simulink model "14_bus"  (R2024a)
settings: Solver=VariableStepAuto  StartTime=0.0  StopTime=1  RelTol=1e-3
undefined symbols (not defined in the file): D1, Delta
libraries: spsRMSLib x186, simulink_extras x171, spsThreePhaseVIMeasurementLib x94, spsThreePhaseBreakerLib x62, spsThreePhaseSeriesRLCBranchLib x20, spsThreePhaseSeriesRLCLoadLib x12, spsThreePhaseSourceLib x5, spsLoadFlowBusLib x5, spsStairGeneratorLib x5, spsThreePhaseTransformerTwoWindingsLib x5, spsThreePhaseFaultLib x5, sps_lib x1
(part 4 of 6)

== system 14_bus/Subsystem14/Subsystem22 ==
  Iabc1 : Inport
  Constant : Constant  Value=2  OutDataTypeStr=boolean
  Constant1 : Constant  Value=0  OutDataTypeStr=boolean
  Data Type Conversion : DataTypeConversion  OutDataTypeStr=double  SaturateOnIntegerOverflow=off  RndMeth=Floor
  Demux : Demux  Outputs=3
  Logical Operator : Logic  Inputs=3  AllPortsSameDT=off  OutDataTypeStr=boolean
  RMS : spsRMSLib/RMS  TrueRMS=on  Freq=60  RMSInit=120  Ts=0
  RMS1 : spsRMSLib/RMS  TrueRMS=on  Freq=60  RMSInit=120  Ts=0
  RMS2 : spsRMSLib/RMS  TrueRMS=on  Freq=60  RMSInit=120  Ts=0
  Relational Operator : RelationalOperator  Operator=>  OutDataTypeStr=boolean  RndMeth=Simplest  InputSameDT=off
  Relational Operator1 : RelationalOperator  Operator=>  OutDataTypeStr=boolean  RndMeth=Simplest  InputSameDT=off
  Relational Operator2 : RelationalOperator  Operator=>  OutDataTypeStr=boolean  RndMeth=Simplest  InputSameDT=off
  S-R Flip-Flop : simulink_extras/Flip Flops/S-R Flip-Flop  initial_condition=0
  S-R Flip-Flop1 : simulink_extras/Flip Flops/S-R Flip-Flop  initial_condition=0
  S-R Flip-Flop2 : simulink_extras/Flip Flops/S-R Flip-Flop  initial_condition=0
  Terminator : Terminator
  Terminator1 : Terminator
  Terminator2 : Terminator
  Out1 : Outport
  wires:
  Data Type Conversion/1 -> Out1/1
  Relational Operator/1 -> S-R Flip-Flop/1
  Constant1/1 -> S-R Flip-Flop/2, S-R Flip-Flop1/2, S-R Flip-Flop2/2
  RMS/1 -> Relational Operator/1
  S-R Flip-Flop1/2 -> Terminator1/1
  S-R Flip-Flop/2 -> Terminator/1
  S-R Flip-Flop2/2 -> Terminator2/1
  Iabc1/1 -> Demux/1
  Logical Operator/1 -> Data Type Conversion/1
  Constant/1 -> Relational Operator/2, Relational Operator1/2, Relational Operator2/2
  S-R Flip-Flop2/1 -> Logical Operator/3
  Relational Operator1/1 -> S-R Flip-Flop1/1
  S-R Flip-Flop/1 -> Logical Operator/1
  S-R Flip-Flop1/1 -> Logical Operator/2
  Relational Operator2/1 -> S-R Flip-Flop2/1
  Demux/1 -> RMS/1
  RMS2/1 -> Relational Operator1/1
  Demux/2 -> RMS2/1
  RMS1/1 -> Relational Operator2/1
  Demux/3 -> RMS1/1

== system 14_bus/Subsystem15/Subsystem8 ==
  Iabc1 : Inport
  Constant : Constant  Value=2  OutDataTypeStr=boolean
  Constant1 : Constant  Value=0  OutDataTypeStr=boolean
  Data Type Conversion : DataTypeConversion  OutDataTypeStr=double  SaturateOnIntegerOverflow=off  RndMeth=Floor
  Demux : Demux  Outputs=3
  Logical Operator : Logic  Inputs=3  AllPortsSameDT=off  OutDataTypeStr=boolean
  RMS : spsRMSLib/RMS  TrueRMS=on  Freq=60  RMSInit=120  Ts=0
  RMS1 : spsRMSLib/RMS  TrueRMS=on  Freq=60  RMSInit=120  Ts=0
  RMS2 : spsRMSLib/RMS  TrueRMS=on  Freq=60  RMSInit=120  Ts=0
  Relational Operator : RelationalOperator  Operator=>  OutDataTypeStr=boolean  RndMeth=Simplest  InputSameDT=off
  Relational Operator1 : RelationalOperator  Operator=>  OutDataTypeStr=boolean  RndMeth=Simplest  InputSameDT=off
  Relational Operator2 : RelationalOperator  Operator=>  OutDataTypeStr=boolean  RndMeth=Simplest  InputSameDT=off
  S-R Flip-Flop : simulink_extras/Flip Flops/S-R Flip-Flop  initial_condition=0
  S-R Flip-Flop1 : simulink_extras/Flip Flops/S-R Flip-Flop  initial_condition=0
  S-R Flip-Flop2 : simulink_extras/Flip Flops/S-R Flip-Flop  initial_condition=0
  Terminator : Terminator
  Terminator1 : Terminator
  Terminator2 : Terminator
  Out1 : Outport
  wires:
  Data Type Conversion/1 -> Out1/1
  Relational Operator/1 -> S-R Flip-Flop/1
  Constant1/1 -> S-R Flip-Flop/2, S-R Flip-Flop1/2, S-R Flip-Flop2/2
  RMS/1 -> Relational Operator/1
  S-R Flip-Flop1/2 -> Terminator1/1
  S-R Flip-Flop/2 -> Terminator/1
  S-R Flip-Flop2/2 -> Terminator2/1
  Iabc1/1 -> Demux/1
  Logical Operator/1 -> Data Type Conversion/1
  Constant/1 -> Relational Operator/2, Relational Operator1/2, Relational Operator2/2
  S-R Flip-Flop2/1 -> Logical Operator/3
  Relational Operator1/1 -> S-R Flip-Flop1/1
  S-R Flip-Flop/1 -> Logical Operator/1
  S-R Flip-Flop1/1 -> Logical Operator/2
  Relational Operator2/1 -> S-R Flip-Flop2/1
  Demux/1 -> RMS/1
  RMS1/1 -> Relational Operator1/1
  Demux/2 -> RMS1/1
  RMS2/1 -> Relational Operator2/1
  Demux/3 -> RMS2/1

== system 14_bus/Subsystem16/Subsystem15 ==
  Iabc1 : Inport
  Constant : Constant  Value=2  OutDataTypeStr=boolean
  Constant1 : Constant  Value=0  OutDataTypeStr=boolean
  Data Type Conversion : DataTypeConversion  OutDataTypeStr=double  SaturateOnIntegerOverflow=off  RndMeth=Floor
  Demux : Demux  Outputs=3
  Logical Operator : Logic  Inputs=3  AllPortsSameDT=off  OutDataTypeStr=boolean
  RMS : spsRMSLib/RMS  TrueRMS=on  Freq=60  RMSInit=120  Ts=0
  RMS1 : spsRMSLib/RMS  TrueRMS=on  Freq=60  RMSInit=120  Ts=0
  RMS2 : spsRMSLib/RMS  TrueRMS=on  Freq=60  RMSInit=120  Ts=0
  Relational Operator : RelationalOperator  Operator=>  OutDataTypeStr=boolean  RndMeth=Simplest  InputSameDT=off
  Relational Operator1 : RelationalOperator  Operator=>  OutDataTypeStr=boolean  RndMeth=Simplest  InputSameDT=off
  Relational Operator2 : RelationalOperator  Operator=>  OutDataTypeStr=boolean  RndMeth=Simplest  InputSameDT=off
  S-R Flip-Flop : simulink_extras/Flip Flops/S-R Flip-Flop  initial_condition=0
  S-R Flip-Flop1 : simulink_extras/Flip Flops/S-R Flip-Flop  initial_condition=0
  S-R Flip-Flop2 : simulink_extras/Flip Flops/S-R Flip-Flop  initial_condition=0
  Terminator : Terminator
  Terminator1 : Terminator
  Terminator2 : Terminator
  Out1 : Outport
  wires:
  Data Type Conversion/1 -> Out1/1
  Relational Operator/1 -> S-R Flip-Flop/1
  Constant1/1 -> S-R Flip-Flop/2, S-R Flip-Flop1/2, S-R Flip-Flop2/2
  RMS/1 -> Relational Operator/1
  S-R Flip-Flop1/2 -> Terminator1/1
  S-R Flip-Flop/2 -> Terminator/1
  S-R Flip-Flop2/2 -> Terminator2/1
  Iabc1/1 -> Demux/1
  Logical Operator/1 -> Data Type Conversion/1
  Constant/1 -> Relational Operator/2, Relational Operator1/2, Relational Operator2/2
  S-R Flip-Flop2/1 -> Logical Operator/3
  Relational Operator1/1 -> S-R Flip-Flop1/1
  S-R Flip-Flop/1 -> Logical Operator/1
  S-R Flip-Flop1/1 -> Logical Operator/2
  Relational Operator2/1 -> S-R Flip-Flop2/1
  Demux/1 -> RMS/1
  RMS1/1 -> Relational Operator1/1
  Demux/2 -> RMS1/1
  ? -> Relational Operator2/1
  Demux/3 -> RMS2/1

== system 14_bus/Subsystem17/Subsystem1 ==
  Iabc1 : Inport
  Constant : Constant  Value=2  OutDataTypeStr=boolean
  Constant1 : Constant  Value=0  OutDataTypeStr=boolean
  Data Type Conversion : DataTypeConversion  OutDataTypeStr=double  SaturateOnIntegerOverflow=off  RndMeth=Floor
  Demux : Demux  Outputs=3
  Logical Operator : Logic  Inputs=3  AllPortsSameDT=off  OutDataTypeStr=boolean
  RMS : spsRMSLib/RMS  TrueRMS=on  Freq=60  RMSInit=120  Ts=0
  RMS1 : spsRMSLib/RMS  TrueRMS=on  Freq=60  RMSInit=120  Ts=0
  RMS2 : spsRMSLib/RMS  TrueRMS=on  Freq=60  RMSInit=120  Ts=0
  Relational Operator : RelationalOperator  Operator=>  OutDataTypeStr=boolean  RndMeth=Simplest  InputSameDT=off
  Relational Operator1 : RelationalOperator  Operator=>  OutDataTypeStr=boolean  RndMeth=Simplest  InputSameDT=off
  Relational Operator2 : RelationalOperator  Operator=>  OutDataTypeStr=boolean  RndMeth=Simplest  InputSameDT=off
  S-R Flip-Flop : simulink_extras/Flip Flops/S-R Flip-Flop  initial_condition=0
  S-R Flip-Flop1 : simulink_extras/Flip Flops/S-R Flip-Flop  initial_condition=0
  S-R Flip-Flop2 : simulink_extras/Flip Flops/S-R Flip-Flop  initial_condition=0
  Terminator : Terminator
  Terminator1 : Terminator
  Terminator2 : Terminator
  Out1 : Outport
  wires:
  Data Type Conversion/1 -> Out1/1
  Relational Operator/1 -> S-R Flip-Flop/1
  Constant1/1 -> S-R Flip-Flop/2, S-R Flip-Flop1/2, S-R Flip-Flop2/2
  RMS/1 -> Relational Operator/1
  S-R Flip-Flop1/2 -> Terminator1/1
  S-R Flip-Flop/2 -> Terminator/1
  S-R Flip-Flop2/2 -> Terminator2/1
  Iabc1/1 -> Demux/1
  Logical Operator/1 -> Data Type Conversion/1
  Constant/1 -> Relational Operator/2, Relational Operator1/2, Relational Operator2/2
  S-R Flip-Flop2/1 -> Logical Operator/3
  Relational Operator1/1 -> S-R Flip-Flop1/1
  S-R Flip-Flop/1 -> Logical Operator/1
  S-R Flip-Flop1/1 -> Logical Operator/2
  Relational Operator2/1 -> S-R Flip-Flop2/1
  Demux/1 -> RMS/1
  RMS1/1 -> Relational Operator1/1
  Demux/2 -> RMS1/1
  RMS2/1 -> Relational Operator2/1
  Demux/3 -> RMS2/1

== system 14_bus/Subsystem18/Subsystem1 ==
  Iabc1 : Inport
  Constant : Constant  Value=2  OutDataTypeStr=boolean
  Constant1 : Constant  Value=0  OutDataTypeStr=boolean
  Data Type Conversion : DataTypeConversion  OutDataTypeStr=double  SaturateOnIntegerOverflow=off  RndMeth=Floor
  Demux : Demux  Outputs=3
  Logical Operator : Logic  Inputs=3  AllPortsSameDT=off  OutDataTypeStr=boolean
  RMS : spsRMSLib/RMS  TrueRMS=on  Freq=60  RMSInit=120  Ts=0
  RMS1 : spsRMSLib/RMS  TrueRMS=on  Freq=60  RMSInit=120  Ts=0
  RMS2 : spsRMSLib/RMS  TrueRMS=on  Freq=60  RMSInit=120  Ts=0
  Relational Operator : RelationalOperator  Operator=>  OutDataTypeStr=boolean  RndMeth=Simplest  InputSameDT=off
  Relational Operator1 : RelationalOperator  Operator=>  OutDataTypeStr=boolean  RndMeth=Simplest  InputSameDT=off
  Relational Operator2 : RelationalOperator  Operator=>  OutDataTypeStr=boolean  RndMeth=Simplest  InputSameDT=off
  S-R Flip-Flop : simulink_extras/Flip Flops/S-R Flip-Flop  initial_condition=0
  S-R Flip-Flop1 : simulink_extras/Flip Flops/S-R Flip-Flop  initial_condition=0
  S-R Flip-Flop2 : simulink_extras/Flip Flops/S-R Flip-Flop  initial_condition=0
  Terminator : Terminator
  Terminator1 : Terminator
  Terminator2 : Terminator
  Out1 : Outport
  wires:
  Data Type Conversion/1 -> Out1/1
  Relational Operator/1 -> S-R Flip-Flop/1
  Constant1/1 -> S-R Flip-Flop/2, S-R Flip-Flop1/2, S-R Flip-Flop2/2
  RMS/1 -> Relational Operator/1
  S-R Flip-Flop1/2 -> Terminator1/1
  S-R Flip-Flop/2 -> Terminator/1
  S-R Flip-Flop2/2 -> Terminator2/1
  Iabc1/1 -> Demux/1
  Logical Operator/1 -> Data Type Conversion/1
  Constant/1 -> Relational Operator/2, Relational Operator1/2, Relational Operator2/2
  S-R Flip-Flop2/1 -> Logical Operator/3
  Relational Operator1/1 -> S-R Flip-Flop1/1
  S-R Flip-Flop/1 -> Logical Operator/1
  S-R Flip-Flop1/1 -> Logical Operator/2
  Relational Operator2/1 -> S-R Flip-Flop2/1
  Demux/1 -> RMS/1
  RMS1/1 -> Relational Operator1/1
  Demux/2 -> RMS1/1
  RMS2/1 -> Relational Operator2/1
  Demux/3 -> RMS2/1

== system 14_bus/Subsystem19/Subsystem21 ==
  Iabc1 : Inport
  Constant : Constant  Value=2  OutDataTypeStr=boolean
  Constant1 : Constant  Value=0  OutDataTypeStr=boolean
  Data Type Conversion : DataTypeConversion  OutDataTypeStr=double  SaturateOnIntegerOverflow=off  RndMeth=Floor
  Demux : Demux  Outputs=3
  Logical Operator : Logic  Inputs=3  AllPortsSameDT=off  OutDataTypeStr=boolean
  RMS : spsRMSLib/RMS  TrueRMS=on  Freq=60  RMSInit=120  Ts=0
  RMS1 : spsRMSLib/RMS  TrueRMS=on  Freq=60  RMSInit=120  Ts=0
  RMS2 : spsRMSLib/RMS  TrueRMS=on  Freq=60  RMSInit=120  Ts=0
  Relational Operator : RelationalOperator  Operator=>  OutDataTypeStr=boolean  RndMeth=Simplest  InputSameDT=off
  Relational Operator1 : RelationalOperator  Operator=>  OutDataTypeStr=boolean  RndMeth=Simplest  InputSameDT=off
  Relational Operator2 : RelationalOperator  Operator=>  OutDataTypeStr=boolean  RndMeth=Simplest  InputSameDT=off
  S-R Flip-Flop : simulink_extras/Flip Flops/S-R Flip-Flop  initial_condition=0
  S-R Flip-Flop1 : simulink_extras/Flip Flops/S-R Flip-Flop  initial_condition=0
  S-R Flip-Flop2 : simulink_extras/Flip Flops/S-R Flip-Flop  initial_condition=0
  Terminator : Terminator
  Terminator1 : Terminator
  Terminator2 : Terminator
  Out1 : Outport
  wires:
  Data Type Conversion/1 -> Out1/1
  Relational Operator/1 -> S-R Flip-Flop/1
  Constant1/1 -> S-R Flip-Flop/2, S-R Flip-Flop1/2, S-R Flip-Flop2/2
  RMS/1 -> Relational Operator/1
  S-R Flip-Flop1/2 -> Terminator1/1
  S-R Flip-Flop/2 -> Terminator/1
  S-R Flip-Flop2/2 -> Terminator2/1
  Iabc1/1 -> Demux/1
  Logical Operator/1 -> Data Type Conversion/1
  Constant/1 -> Relational Operator/2, Relational Operator1/2, Relational Operator2/2
  S-R Flip-Flop2/1 -> Logical Operator/3
  Relational Operator1/1 -> S-R Flip-Flop1/1
  S-R Flip-Flop/1 -> Logical Operator/1
  S-R Flip-Flop1/1 -> Logical Operator/2
  Relational Operator2/1 -> S-R Flip-Flop2/1
  Demux/1 -> RMS/1
  RMS2/1 -> Relational Operator1/1
  Demux/2 -> RMS2/1
  RMS1/1 -> Relational Operator2/1
  Demux/3 -> RMS1/1

== system 14_bus/Subsystem2/Subsystem1 ==
  Iabc1 : Inport
  Constant : Constant  Value=2  OutDataTypeStr=boolean
  Constant1 : Constant  Value=0  OutDataTypeStr=boolean
  Data Type Conversion : DataTypeConversion  OutDataTypeStr=double  SaturateOnIntegerOverflow=off  RndMeth=Floor
  Demux : Demux  Outputs=3
  Logical Operator : Logic  Inputs=3  AllPortsSameDT=off  OutDataTypeStr=boolean
  RMS : spsRMSLib/RMS  TrueRMS=on  Freq=60  RMSInit=120  Ts=0
  RMS1 : spsRMSLib/RMS  TrueRMS=on  Freq=60  RMSInit=120  Ts=0
  RMS2 : spsRMSLib/RMS  TrueRMS=on  Freq=60  RMSInit=120  Ts=0
  Relational Operator : RelationalOperator  Operator=>  OutDataTypeStr=boolean  RndMeth=Simplest  InputSameDT=off
  Relational Operator1 : RelationalOperator  Operator=>  OutDataTypeStr=boolean  RndMeth=Simplest  InputSameDT=off
  Relational Operator2 : RelationalOperator  Operator=>  OutDataTypeStr=boolean  RndMeth=Simplest  InputSameDT=off
  S-R Flip-Flop : simulink_extras/Flip Flops/S-R Flip-Flop  initial_condition=0
  S-R Flip-Flop1 : simulink_extras/Flip Flops/S-R Flip-Flop  initial_condition=0
  S-R Flip-Flop2 : simulink_extras/Flip Flops/S-R Flip-Flop  initial_condition=0
  Terminator : Terminator
  Terminator1 : Terminator
  Terminator2 : Terminator
  Out1 : Outport
  wires:
  Data Type Conversion/1 -> Out1/1
  Relational Operator/1 -> S-R Flip-Flop/1
  Constant1/1 -> S-R Flip-Flop/2, S-R Flip-Flop1/2, S-R Flip-Flop2/2
  RMS2/1 -> Relational Operator/1
  S-R Flip-Flop1/2 -> Terminator1/1
  S-R Flip-Flop/2 -> Terminator/1
  S-R Flip-Flop2/2 -> Terminator2/1
  Iabc1/1 -> Demux/1
  Logical Operator/1 -> Data Type Conversion/1
  Constant/1 -> Relational Operator/2, Relational Operator1/2, Relational Operator2/2
  S-R Flip-Flop2/1 -> Logical Operator/3
  Relational Operator1/1 -> S-R Flip-Flop1/1
  S-R Flip-Flop/1 -> Logical Operator/1
  S-R Flip-Flop1/1 -> Logical Operator/2
  Relational Operator2/1 -> S-R Flip-Flop2/1
  Demux/1 -> RMS2/1
  RMS1/1 -> Relational Operator1/1
  Demux/2 -> RMS1/1
  RMS/1 -> Relational Operator2/1
  Demux/3 -> RMS/1

== system 14_bus/Subsystem20/Subsystem1 ==
  Iabc1 : Inport
  Constant : Constant  Value=2  OutDataTypeStr=boolean
  Constant1 : Constant  Value=0  OutDataTypeStr=boolean
  Data Type Conversion : DataTypeConversion  OutDataTypeStr=double  SaturateOnIntegerOverflow=off  RndMeth=Floor
  Demux : Demux  Outputs=3
  Logical Operator : Logic  Inputs=3  AllPortsSameDT=off  OutDataTypeStr=boolean
  RMS : spsRMSLib/RMS  TrueRMS=on  Freq=60  RMSInit=120  Ts=0
  RMS1 : spsRMSLib/RMS  TrueRMS=on  Freq=60  RMSInit=120  Ts=0
  RMS2 : spsRMSLib/RMS  TrueRMS=on  Freq=60  RMSInit=120  Ts=0
  Relational Operator : RelationalOperator  Operator=>  OutDataTypeStr=boolean  RndMeth=Simplest  InputSameDT=off
  Relational Operator1 : RelationalOperator  Operator=>  OutDataTypeStr=boolean  RndMeth=Simplest  InputSameDT=off
  Relational Operator2 : RelationalOperator  Operator=>  OutDataTypeStr=boolean  RndMeth=Simplest  InputSameDT=off
  S-R Flip-Flop : simulink_extras/Flip Flops/S-R Flip-Flop  initial_condition=0
  S-R Flip-Flop1 : simulink_extras/Flip Flops/S-R Flip-Flop  initial_condition=0
  S-R Flip-Flop2 : simulink_extras/Flip Flops/S-R Flip-Flop  initial_condition=0
  Terminator : Terminator
  Terminator1 : Terminator
  Terminator2 : Terminator
  Out1 : Outport
  wires:
  Data Type Conversion/1 -> Out1/1
  Relational Operator/1 -> S-R Flip-Flop/1
  Constant1/1 -> S-R Flip-Flop/2, S-R Flip-Flop1/2, S-R Flip-Flop2/2
  RMS/1 -> Relational Operator/1
  S-R Flip-Flop1/2 -> Terminator1/1
  S-R Flip-Flop/2 -> Terminator/1
  S-R Flip-Flop2/2 -> Terminator2/1
  Iabc1/1 -> Demux/1
  Logical Operator/1 -> Data Type Conversion/1
  Constant/1 -> Relational Operator/2, Relational Operator1/2, Relational Operator2/2
  S-R Flip-Flop2/1 -> Logical Operator/3
  Relational Operator1/1 -> S-R Flip-Flop1/1
  S-R Flip-Flop/1 -> Logical Operator/1
  S-R Flip-Flop1/1 -> Logical Operator/2
  Relational Operator2/1 -> S-R Flip-Flop2/1
  Demux/1 -> RMS/1
  RMS1/1 -> Relational Operator1/1
  Demux/2 -> RMS1/1
  RMS2/1 -> Relational Operator2/1
  Demux/3 -> RMS2/1

== system 14_bus/Subsystem21/Subsystem23 ==
  Iabc1 : Inport
  Constant : Constant  Value=2  OutDataTypeStr=boolean
  Constant1 : Constant  Value=0  OutDataTypeStr=boolean
  Data Type Conversion : DataTypeConversion  OutDataTypeStr=double  SaturateOnIntegerOverflow=off  RndMeth=Floor
  Demux : Demux  Outputs=3
  Logical Operator : Logic  Inputs=3  AllPortsSameDT=off  OutDataTypeStr=boolean
  RMS : spsRMSLib/RMS  TrueRMS=on  Freq=60  RMSInit=120  Ts=0
  RMS1 : spsRMSLib/RMS  TrueRMS=on  Freq=60  RMSInit=120  Ts=0
  RMS2 : spsRMSLib/RMS  TrueRMS=on  Freq=60  RMSInit=120  Ts=0
  Relational Operator : RelationalOperator  Operator=>  OutDataTypeStr=boolean  RndMeth=Simplest  InputSameDT=off
  Relational Operator1 : RelationalOperator  Operator=>  OutDataTypeStr=boolean  RndMeth=Simplest  InputSameDT=off
  Relational Operator2 : RelationalOperator  Operator=>  OutDataTypeStr=boolean  RndMeth=Simplest  InputSameDT=off
  S-R Flip-Flop : simulink_extras/Flip Flops/S-R Flip-Flop  initial_condition=0
  S-R Flip-Flop1 : simulink_extras/Flip Flops/S-R Flip-Flop  initial_condition=0
  S-R Flip-Flop2 : simulink_extras/Flip Flops/S-R Flip-Flop  initial_condition=0
  Terminator : Terminator
  Terminator1 : Terminator
  Terminator2 : Terminator
  Out1 : Outport
  wires:
  Data Type Conversion/1 -> Out1/1
  Relational Operator/1 -> S-R Flip-Flop/1
  Constant1/1 -> S-R Flip-Flop/2, S-R Flip-Flop1/2, S-R Flip-Flop2/2
  RMS1/1 -> Relational Operator/1
  S-R Flip-Flop1/2 -> Terminator1/1
  S-R Flip-Flop/2 -> Terminator/1
  S-R Flip-Flop2/2 -> Terminator2/1
  Iabc1/1 -> Demux/1
  Logical Operator/1 -> Data Type Conversion/1
  Constant/1 -> Relational Operator/2, Relational Operator1/2, Relational Operator2/2
  S-R Flip-Flop2/1 -> Logical Operator/3
  Relational Operator1/1 -> S-R Flip-Flop1/1
  S-R Flip-Flop/1 -> Logical Operator/1
  S-R Flip-Flop1/1 -> Logical Operator/2
  Relational Operator2/1 -> S-R Flip-Flop2/1
  Demux/1 -> RMS1/1
  RMS2/1 -> Relational Operator1/1
  Demux/2 -> RMS2/1
  RMS/1 -> Relational Operator2/1
  Demux/3 -> RMS/1

== system 14_bus/Subsystem22/Subsystem1 ==
  Iabc1 : Inport
  Constant : Constant  Value=2  OutDataTypeStr=boolean
  Constant1 : Constant  Value=0  OutDataTypeStr=boolean
  Data Type Conversion : DataTypeConversion  OutDataTypeStr=double  SaturateOnIntegerOverflow=off  RndMeth=Floor
  Demux : Demux  Outputs=3
  Logical Operator : Logic  Inputs=3  AllPortsSameDT=off  OutDataTypeStr=boolean
  RMS : spsRMSLib/RMS  TrueRMS=on  Freq=60  RMSInit=120  Ts=0
  RMS1 : spsRMSLib/RMS  TrueRMS=on  Freq=60  RMSInit=120  Ts=0
  RMS2 : spsRMSLib/RMS  TrueRMS=on  Freq=60  RMSInit=120  Ts=0
  Relational Operator : RelationalOperator  Operator=>  OutDataTypeStr=boolean  RndMeth=Simplest  InputSameDT=off
  Relational Operator1 : RelationalOperator  Operator=>  OutDataTypeStr=boolean  RndMeth=Simplest  InputSameDT=off
  Relational Operator2 : RelationalOperator  Operator=>  OutDataTypeStr=boolean  RndMeth=Simplest  InputSameDT=off
  S-R Flip-Flop : simulink_extras/Flip Flops/S-R Flip-Flop  initial_condition=0
  S-R Flip-Flop1 : simulink_extras/Flip Flops/S-R Flip-Flop  initial_condition=0
  S-R Flip-Flop2 : simulink_extras/Flip Flops/S-R Flip-Flop  initial_condition=0
  Terminator : Terminator
  Terminator1 : Terminator
  Terminator2 : Terminator
  Out1 : Outport
  wires:
  Data Type Conversion/1 -> Out1/1
  Relational Operator/1 -> S-R Flip-Flop/1
  Constant1/1 -> S-R Flip-Flop/2, S-R Flip-Flop1/2, S-R Flip-Flop2/2
  RMS/1 -> Relational Operator/1
  S-R Flip-Flop1/2 -> Terminator1/1
  S-R Flip-Flop/2 -> Terminator/1
  S-R Flip-Flop2/2 -> Terminator2/1
  Iabc1/1 -> Demux/1
  Logical Operator/1 -> Data Type Conversion/1
  Constant/1 -> Relational Operator/2, Relational Operator1/2, Relational Operator2/2
  S-R Flip-Flop2/1 -> Logical Operator/3
  Relational Operator1/1 -> S-R Flip-Flop1/1
  S-R Flip-Flop/1 -> Logical Operator/1
  S-R Flip-Flop1/1 -> Logical Operator/2
  Relational Operator2/1 -> S-R Flip-Flop2/1
  Demux/1 -> RMS/1
  RMS1/1 -> Relational Operator1/1
  Demux/2 -> RMS1/1
  RMS2/1 -> Relational Operator2/1
  Demux/3 -> RMS2/1

== system 14_bus/Subsystem23/Subsystem24 ==
  Iabc1 : Inport
  Constant : Constant  Value=2  OutDataTypeStr=boolean
  Constant1 : Constant  Value=0  OutDataTypeStr=boolean
  Data Type Conversion : DataTypeConversion  OutDataTypeStr=double  SaturateOnIntegerOverflow=off  RndMeth=Floor
  Demux : Demux  Outputs=3
  Logical Operator : Logic  Inputs=3  AllPortsSameDT=off  OutDataTypeStr=boolean
  RMS : spsRMSLib/RMS  TrueRMS=on  Freq=60  RMSInit=120  Ts=0
  RMS1 : spsRMSLib/RMS  TrueRMS=on  Freq=60  RMSInit=120  Ts=0
  RMS2 : spsRMSLib/RMS  TrueRMS=on  Freq=60  RMSInit=120  Ts=0
  Relational Operator : RelationalOperator  Operator=>  OutDataTypeStr=boolean  RndMeth=Simplest  InputSameDT=off
  Relational Operator1 : RelationalOperator  Operator=>  OutDataTypeStr=boolean  RndMeth=Simplest  InputSameDT=off
  Relational Operator2 : RelationalOperator  Operator=>  OutDataTypeStr=boolean  RndMeth=Simplest  InputSameDT=off
  S-R Flip-Flop : simulink_extras/Flip Flops/S-R Flip-Flop  initial_condition=0
  S-R Flip-Flop1 : simulink_extras/Flip Flops/S-R Flip-Flop  initial_condition=0
  S-R Flip-Flop2 : simulink_extras/Flip Flops/S-R Flip-Flop  initial_condition=0
  Terminator : Terminator
  Terminator1 : Terminator
  Terminator2 : Terminator
  Out1 : Outport
  wires:
  Data Type Conversion/1 -> Out1/1
  Relational Operator/1 -> S-R Flip-Flop/1
  Constant1/1 -> S-R Flip-Flop/2, S-R Flip-Flop1/2, S-R Flip-Flop2/2
  RMS/1 -> Relational Operator/1
  S-R Flip-Flop1/2 -> Terminator1/1
  S-R Flip-Flop/2 -> Terminator/1
  S-R Flip-Flop2/2 -> Terminator2/1
  Iabc1/1 -> Demux/1
  Logical Operator/1 -> Data Type Conversion/1
  Constant/1 -> Relational Operator/2, Relational Operator1/2, Relational Operator2/2
  S-R Flip-Flop2/1 -> Logical Operator/3
  Relational Operator1/1 -> S-R Flip-Flop1/1
  S-R Flip-Flop/1 -> Logical Operator/1
  S-R Flip-Flop1/1 -> Logical Operator/2
  Relational Operator2/1 -> S-R Flip-Flop2/1
  Demux/1 -> RMS/1
  RMS1/1 -> Relational Operator1/1
  Demux/2 -> RMS1/1
  RMS2/1 -> Relational Operator2/1
  Demux/3 -> RMS2/1

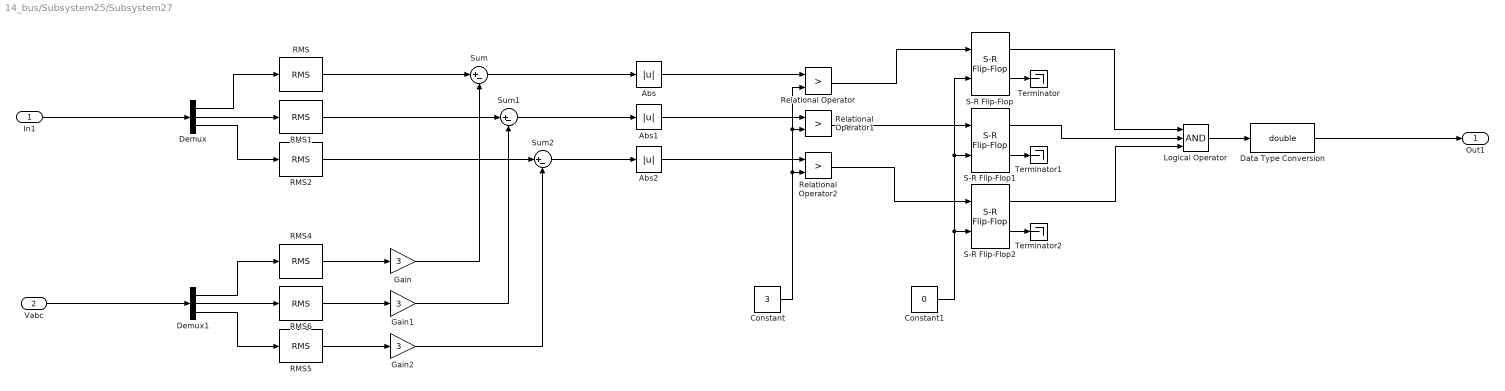
== system 14_bus/Subsystem25/Subsystem27 ==
  In1 : Inport
  Vabc : Inport  Port=2
  Abs : Abs  SaturateOnIntegerOverflow=off
  Abs1 : Abs  SaturateOnIntegerOverflow=off
  Abs2 : Abs  SaturateOnIntegerOverflow=off
  Constant : Constant  Value=3  OutDataTypeStr=boolean
  Constant1 : Constant  Value=0  OutDataTypeStr=boolean
  Data Type Conversion : DataTypeConversion  OutDataTypeStr=double  SaturateOnIntegerOverflow=off  RndMeth=Floor
  Demux : Demux  Outputs=3
  Demux1 : Demux  Outputs=3
  Gain : Gain  Gain=3
  Gain1 : Gain  Gain=3
  Gain2 : Gain  Gain=3
  Logical Operator : Logic  Inputs=3  AllPortsSameDT=off  OutDataTypeStr=boolean
  RMS{,1..2,4..6} (6 alike) : spsRMSLib/RMS  TrueRMS=on  Freq=60  RMSInit=120  Ts=0
  Relational Operator : RelationalOperator  Operator=>  OutDataTypeStr=boolean  RndMeth=Simplest  InputSameDT=off
  Relational Operator1 : RelationalOperator  Operator=>  OutDataTypeStr=boolean  RndMeth=Simplest  InputSameDT=off
  Relational Operator2 : RelationalOperator  Operator=>  OutDataTypeStr=boolean  RndMeth=Simplest  InputSameDT=off
  S-R Flip-Flop : simulink_extras/Flip Flops/S-R Flip-Flop  initial_condition=0
  S-R Flip-Flop1 : simulink_extras/Flip Flops/S-R Flip-Flop  initial_condition=0
  S-R Flip-Flop2 : simulink_extras/Flip Flops/S-R Flip-Flop  initial_condition=0
  Sum : Sum  Inputs=|+-
  Sum1 : Sum  Inputs=|+-
  Sum2 : Sum  Inputs=|+-
  Terminator : Terminator
  Terminator1 : Terminator
  Terminator2 : Terminator
  Out1 : Outport
  wires:
  Sum1/1 -> Abs1/1
  RMS6/1 -> Gain1/1
  Sum/1 -> Abs/1
  RMS2/1 -> Sum2/1
  Abs/1 -> Relational Operator/1
  Relational Operator/1 -> S-R Flip-Flop/1
  Constant/1 -> Relational Operator/2, Relational Operator1/2, Relational Operator2/2
  RMS5/1 -> Gain2/1
  S-R Flip-Flop1/2 -> Terminator1/1
  In1/1 -> Demux/1
  Demux1/3 -> RMS5/1
  RMS1/1 -> Sum1/1
  RMS/1 -> Sum/1
  RMS4/1 -> Gain/1
  Gain2/1 -> Sum2/2
  S-R Flip-Flop2/2 -> Terminator2/1
  Gain/1 -> Sum/2
  Abs2/1 -> Relational Operator2/1
  Demux/3 -> RMS2/1
  Demux1/2 -> RMS6/1
  Data Type Conversion/1 -> Out1/1
  Sum2/1 -> Abs2/1
  Constant1/1 -> S-R Flip-Flop/2, S-R Flip-Flop1/2, S-R Flip-Flop2/2
  Gain1/1 -> Sum1/2
  S-R Flip-Flop/1 -> Logical Operator/1
  Demux/1 -> RMS/1
  Demux1/1 -> RMS4/1
  Demux/2 -> RMS1/1
  S-R Flip-Flop1/1 -> Logical Operator/2
  Relational Operator2/1 -> S-R Flip-Flop2/1
  S-R Flip-Flop/2 -> Terminator/1
  Logical Operator/1 -> Data Type Conversion/1
  S-R Flip-Flop2/1 -> Logical Operator/3
  Relational Operator1/1 -> S-R Flip-Flop1/1
  Abs1/1 -> Relational Operator1/1
  Vabc/1 -> Demux1/1

== system 14_bus/Subsystem26/Subsystem25 ==
  Iabc1 : Inport
  Constant : Constant  Value=2  OutDataTypeStr=boolean
  Constant1 : Constant  Value=0  OutDataTypeStr=boolean
  Data Type Conversion : DataTypeConversion  OutDataTypeStr=double  SaturateOnIntegerOverflow=off  RndMeth=Floor
  Demux : Demux  Outputs=3
  Logical Operator : Logic  Inputs=3  AllPortsSameDT=off  OutDataTypeStr=boolean
  RMS : spsRMSLib/RMS  TrueRMS=on  Freq=60  RMSInit=120  Ts=0
  RMS1 : spsRMSLib/RMS  TrueRMS=on  Freq=60  RMSInit=120  Ts=0
  RMS2 : spsRMSLib/RMS  TrueRMS=on  Freq=60  RMSInit=120  Ts=0
  Relational Operator : RelationalOperator  Operator=>  OutDataTypeStr=boolean  RndMeth=Simplest  InputSameDT=off
  Relational Operator1 : RelationalOperator  Operator=>  OutDataTypeStr=boolean  RndMeth=Simplest  InputSameDT=off
  Relational Operator2 : RelationalOperator  Operator=>  OutDataTypeStr=boolean  RndMeth=Simplest  InputSameDT=off
  S-R Flip-Flop : simulink_extras/Flip Flops/S-R Flip-Flop  initial_condition=0
  S-R Flip-Flop1 : simulink_extras/Flip Flops/S-R Flip-Flop  initial_condition=0
  S-R Flip-Flop2 : simulink_extras/Flip Flops/S-R Flip-Flop  initial_condition=0
  Terminator : Terminator
  Terminator1 : Terminator
  Terminator2 : Terminator
  Out1 : Outport
  wires:
  Data Type Conversion/1 -> Out1/1
  Relational Operator/1 -> S-R Flip-Flop/1
  Constant1/1 -> S-R Flip-Flop/2, S-R Flip-Flop1/2, S-R Flip-Flop2/2
  RMS/1 -> Relational Operator/1
  S-R Flip-Flop1/2 -> Terminator1/1
  S-R Flip-Flop/2 -> Terminator/1
  S-R Flip-Flop2/2 -> Terminator2/1
  Iabc1/1 -> Demux/1
  Logical Operator/1 -> Data Type Conversion/1
  Constant/1 -> Relational Operator/2, Relational Operator1/2, Relational Operator2/2
  S-R Flip-Flop2/1 -> Logical Operator/3
  Relational Operator1/1 -> S-R Flip-Flop1/1
  S-R Flip-Flop/1 -> Logical Operator/1
  S-R Flip-Flop1/1 -> Logical Operator/2
  Relational Operator2/1 -> S-R Flip-Flop2/1
  Demux/1 -> RMS/1
  RMS1/1 -> Relational Operator1/1
  Demux/2 -> RMS1/1
  RMS2/1 -> Relational Operator2/1
  Demux/3 -> RMS2/1

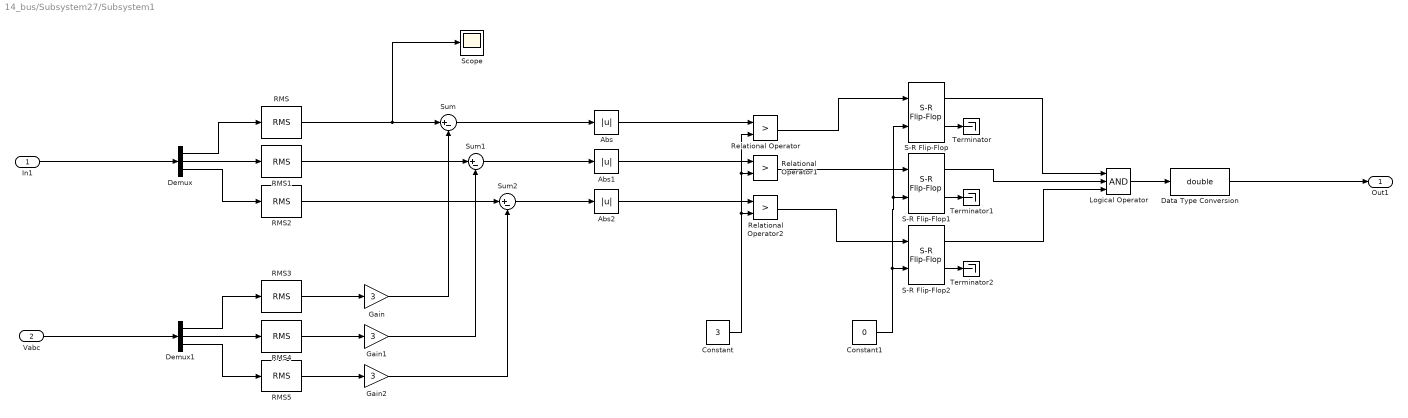
== system 14_bus/Subsystem27/Subsystem1 ==
  In1 : Inport
  Vabc : Inport  Port=2
  Abs : Abs  SaturateOnIntegerOverflow=off
  Abs1 : Abs  SaturateOnIntegerOverflow=off
  Abs2 : Abs  SaturateOnIntegerOverflow=off
  Constant : Constant  Value=3  OutDataTypeStr=boolean
  Constant1 : Constant  Value=0  OutDataTypeStr=boolean
  Data Type Conversion : DataTypeConversion  OutDataTypeStr=double  SaturateOnIntegerOverflow=off  RndMeth=Floor
  Demux : Demux  Outputs=3
  Demux1 : Demux  Outputs=3
  Gain : Gain  Gain=3
  Gain1 : Gain  Gain=3
  Gain2 : Gain  Gain=3
  Logical Operator : Logic  Inputs=3  AllPortsSameDT=off  OutDataTypeStr=boolean
  RMS{,1..5} (6 alike) : spsRMSLib/RMS  TrueRMS=on  Freq=60  RMSInit=120  Ts=0.2
  Relational Operator : RelationalOperator  Operator=>  OutDataTypeStr=boolean  RndMeth=Simplest  InputSameDT=off
  Relational Operator1 : RelationalOperator  Operator=>  OutDataTypeStr=boolean  RndMeth=Simplest  InputSameDT=off
  Relational Operator2 : RelationalOperator  Operator=>  OutDataTypeStr=boolean  RndMeth=Simplest  InputSameDT=off
  S-R Flip-Flop : simulink_extras/Flip Flops/S-R Flip-Flop  initial_condition=0
  S-R Flip-Flop1 : simulink_extras/Flip Flops/S-R Flip-Flop  initial_condition=0
  S-R Flip-Flop2 : simulink_extras/Flip Flops/S-R Flip-Flop  initial_condition=0
  Scope : Scope
  Sum : Sum  Inputs=|+-
  Sum1 : Sum  Inputs=|+-
  Sum2 : Sum  Inputs=|+-
  Terminator : Terminator
  Terminator1 : Terminator
  Terminator2 : Terminator
  Out1 : Outport
  wires:
  Sum1/1 -> Abs1/1
  RMS4/1 -> Gain1/1
  Sum/1 -> Abs/1
  RMS2/1 -> Sum2/1
  Abs/1 -> Relational Operator/1
  Relational Operator/1 -> S-R Flip-Flop/1
  Constant/1 -> Relational Operator/2, Relational Operator1/2, Relational Operator2/2
  RMS5/1 -> Gain2/1
  S-R Flip-Flop1/2 -> Terminator1/1
  In1/1 -> Demux/1
  Demux1/3 -> RMS5/1
  RMS1/1 -> Sum1/1
  RMS/1 -> Scope/1, Sum/1
  RMS3/1 -> Gain/1
  Gain2/1 -> Sum2/2
  S-R Flip-Flop2/2 -> Terminator2/1
  Gain/1 -> Sum/2
  Abs2/1 -> Relational Operator2/1
  Demux/3 -> RMS2/1
  Demux1/2 -> RMS4/1
  Data Type Conversion/1 -> Out1/1
  Sum2/1 -> Abs2/1
  Constant1/1 -> S-R Flip-Flop/2, S-R Flip-Flop1/2, S-R Flip-Flop2/2
  Gain1/1 -> Sum1/2
  S-R Flip-Flop/1 -> Logical Operator/1
  Demux/1 -> RMS/1
  Demux1/1 -> RMS3/1
  Demux/2 -> RMS1/1
  S-R Flip-Flop1/1 -> Logical Operator/2
  Relational Operator2/1 -> S-R Flip-Flop2/1
  S-R Flip-Flop/2 -> Terminator/1
  Logical Operator/1 -> Data Type Conversion/1
  S-R Flip-Flop2/1 -> Logical Operator/3
  Relational Operator1/1 -> S-R Flip-Flop1/1
  Abs1/1 -> Relational Operator1/1
  Vabc/1 -> Demux1/1

== system 14_bus/Subsystem28/Subsystem1 ==
  Iabc1 : Inport
  Constant : Constant  Value=2  OutDataTypeStr=boolean
  Constant1 : Constant  Value=0  OutDataTypeStr=boolean
  Data Type Conversion : DataTypeConversion  OutDataTypeStr=double  SaturateOnIntegerOverflow=off  RndMeth=Floor
  Demux : Demux  Outputs=3
  Logical Operator : Logic  Inputs=3  AllPortsSameDT=off  OutDataTypeStr=boolean
  RMS : spsRMSLib/RMS  TrueRMS=on  Freq=60  RMSInit=120  Ts=0
  RMS1 : spsRMSLib/RMS  TrueRMS=on  Freq=60  RMSInit=120  Ts=0
  RMS2 : spsRMSLib/RMS  TrueRMS=on  Freq=60  RMSInit=120  Ts=0
  Relational Operator : RelationalOperator  Operator=>  OutDataTypeStr=boolean  RndMeth=Simplest  InputSameDT=off
  Relational Operator1 : RelationalOperator  Operator=>  OutDataTypeStr=boolean  RndMeth=Simplest  InputSameDT=off
  Relational Operator2 : RelationalOperator  Operator=>  OutDataTypeStr=boolean  RndMeth=Simplest  InputSameDT=off
  S-R Flip-Flop : simulink_extras/Flip Flops/S-R Flip-Flop  initial_condition=0
  S-R Flip-Flop1 : simulink_extras/Flip Flops/S-R Flip-Flop  initial_condition=0
  S-R Flip-Flop2 : simulink_extras/Flip Flops/S-R Flip-Flop  initial_condition=0
  Terminator : Terminator
  Terminator1 : Terminator
  Terminator2 : Terminator
  Out1 : Outport
  wires:
  Data Type Conversion/1 -> Out1/1
  Relational Operator/1 -> S-R Flip-Flop/1
  Constant1/1 -> S-R Flip-Flop/2, S-R Flip-Flop1/2, S-R Flip-Flop2/2
  RMS/1 -> Relational Operator/1
  S-R Flip-Flop1/2 -> Terminator1/1
  S-R Flip-Flop/2 -> Terminator/1
  S-R Flip-Flop2/2 -> Terminator2/1
  Iabc1/1 -> Demux/1
  Logical Operator/1 -> Data Type Conversion/1
  Constant/1 -> Relational Operator/2, Relational Operator1/2, Relational Operator2/2
  S-R Flip-Flop2/1 -> Logical Operator/3
  Relational Operator1/1 -> S-R Flip-Flop1/1
  S-R Flip-Flop/1 -> Logical Operator/1
  S-R Flip-Flop1/1 -> Logical Operator/2
  Relational Operator2/1 -> S-R Flip-Flop2/1
  Demux/1 -> RMS/1
  RMS1/1 -> Relational Operator1/1
  Demux/2 -> RMS1/1
  RMS2/1 -> Relational Operator2/1
  Demux/3 -> RMS2/1

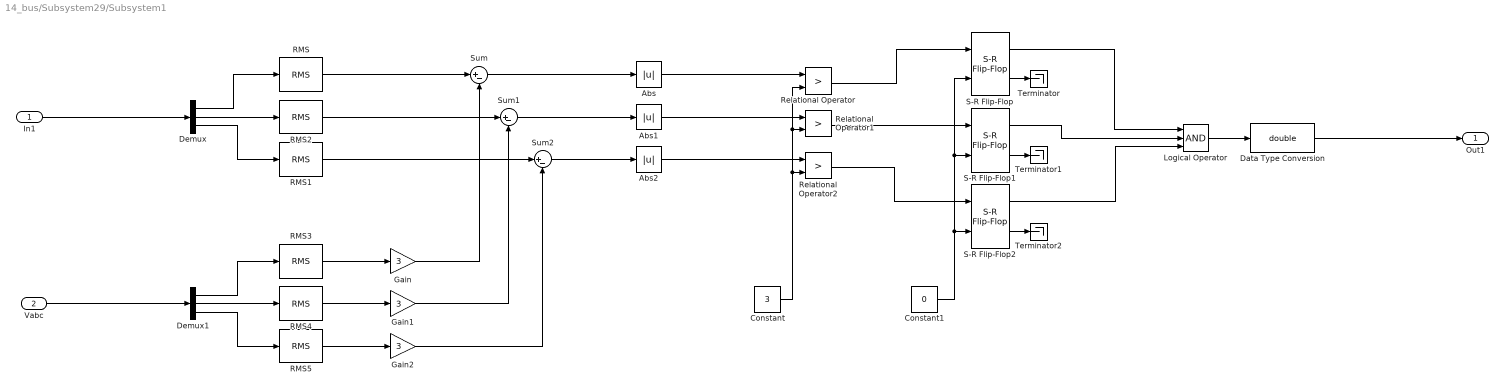
== system 14_bus/Subsystem29/Subsystem1 ==
  In1 : Inport
  Vabc : Inport  Port=2
  Abs : Abs  SaturateOnIntegerOverflow=off
  Abs1 : Abs  SaturateOnIntegerOverflow=off
  Abs2 : Abs  SaturateOnIntegerOverflow=off
  Constant : Constant  Value=3  OutDataTypeStr=boolean
  Constant1 : Constant  Value=0  OutDataTypeStr=boolean
  Data Type Conversion : DataTypeConversion  OutDataTypeStr=double  SaturateOnIntegerOverflow=off  RndMeth=Floor
  Demux : Demux  Outputs=3
  Demux1 : Demux  Outputs=3
  Gain : Gain  Gain=3
  Gain1 : Gain  Gain=3
  Gain2 : Gain  Gain=3
  Logical Operator : Logic  Inputs=3  AllPortsSameDT=off  OutDataTypeStr=boolean
  RMS{,1..5} (6 alike) : spsRMSLib/RMS  TrueRMS=on  Freq=60  RMSInit=120  Ts=0
  Relational Operator : RelationalOperator  Operator=>  OutDataTypeStr=boolean  RndMeth=Simplest  InputSameDT=off
  Relational Operator1 : RelationalOperator  Operator=>  OutDataTypeStr=boolean  RndMeth=Simplest  InputSameDT=off
  Relational Operator2 : RelationalOperator  Operator=>  OutDataTypeStr=boolean  RndMeth=Simplest  InputSameDT=off
  S-R Flip-Flop : simulink_extras/Flip Flops/S-R Flip-Flop  initial_condition=0
  S-R Flip-Flop1 : simulink_extras/Flip Flops/S-R Flip-Flop  initial_condition=0
  S-R Flip-Flop2 : simulink_extras/Flip Flops/S-R Flip-Flop  initial_condition=0
  Sum : Sum  Inputs=|+-
  Sum1 : Sum  Inputs=|+-
  Sum2 : Sum  Inputs=|+-
  Terminator : Terminator
  Terminator1 : Terminator
  Terminator2 : Terminator
  Out1 : Outport
  wires:
  Sum1/1 -> Abs1/1
  RMS4/1 -> Gain1/1
  Sum/1 -> Abs/1
  RMS1/1 -> Sum2/1
  Abs/1 -> Relational Operator/1
  Relational Operator/1 -> S-R Flip-Flop/1
  Constant/1 -> Relational Operator/2, Relational Operator1/2, Relational Operator2/2
  RMS5/1 -> Gain2/1
  S-R Flip-Flop1/2 -> Terminator1/1
  In1/1 -> Demux/1
  Demux1/3 -> RMS5/1
  RMS2/1 -> Sum1/1
  RMS/1 -> Sum/1
  RMS3/1 -> Gain/1
  Gain2/1 -> Sum2/2
  S-R Flip-Flop2/2 -> Terminator2/1
  Gain/1 -> Sum/2
  Abs2/1 -> Relational Operator2/1
  Demux/3 -> RMS1/1
  Demux1/2 -> RMS4/1
  Data Type Conversion/1 -> Out1/1
  Sum2/1 -> Abs2/1
  Constant1/1 -> S-R Flip-Flop/2, S-R Flip-Flop1/2, S-R Flip-Flop2/2
  Gain1/1 -> Sum1/2
  S-R Flip-Flop/1 -> Logical Operator/1
  Demux/1 -> RMS/1
  Demux1/1 -> RMS3/1
  Demux/2 -> RMS2/1
  S-R Flip-Flop1/1 -> Logical Operator/2
  Relational Operator2/1 -> S-R Flip-Flop2/1
  S-R Flip-Flop/2 -> Terminator/1
  Logical Operator/1 -> Data Type Conversion/1
  S-R Flip-Flop2/1 -> Logical Operator/3
  Relational Operator1/1 -> S-R Flip-Flop1/1
  Abs1/1 -> Relational Operator1/1
  Vabc/1 -> Demux1/1

== system 14_bus/Subsystem3/Subsystem16 ==
  Iabc1 : Inport
  Constant : Constant  Value=2  OutDataTypeStr=boolean
  Constant1 : Constant  Value=0  OutDataTypeStr=boolean
  Data Type Conversion : DataTypeConversion  OutDataTypeStr=double  SaturateOnIntegerOverflow=off  RndMeth=Floor
  Demux : Demux  Outputs=3
  Logical Operator : Logic  Inputs=3  AllPortsSameDT=off  OutDataTypeStr=boolean
  RMS : spsRMSLib/RMS  TrueRMS=on  Freq=60  RMSInit=120  Ts=0
  RMS1 : spsRMSLib/RMS  TrueRMS=on  Freq=60  RMSInit=120  Ts=0
  RMS2 : spsRMSLib/RMS  TrueRMS=on  Freq=60  RMSInit=120  Ts=0
  Relational Operator : RelationalOperator  Operator=>  OutDataTypeStr=boolean  RndMeth=Simplest  InputSameDT=off
  Relational Operator1 : RelationalOperator  Operator=>  OutDataTypeStr=boolean  RndMeth=Simplest  InputSameDT=off
  Relational Operator2 : RelationalOperator  Operator=>  OutDataTypeStr=boolean  RndMeth=Simplest  InputSameDT=off
  S-R Flip-Flop : simulink_extras/Flip Flops/S-R Flip-Flop  initial_condition=0
  S-R Flip-Flop1 : simulink_extras/Flip Flops/S-R Flip-Flop  initial_condition=0
  S-R Flip-Flop2 : simulink_extras/Flip Flops/S-R Flip-Flop  initial_condition=0
  Terminator : Terminator
  Terminator1 : Terminator
  Terminator2 : Terminator
  Out1 : Outport
  wires:
  Data Type Conversion/1 -> Out1/1
  Relational Operator/1 -> S-R Flip-Flop/1
  Constant1/1 -> S-R Flip-Flop/2, S-R Flip-Flop1/2, S-R Flip-Flop2/2
  RMS/1 -> Relational Operator/1
  S-R Flip-Flop1/2 -> Terminator1/1
  S-R Flip-Flop/2 -> Terminator/1
  S-R Flip-Flop2/2 -> Terminator2/1
  Iabc1/1 -> Demux/1
  Logical Operator/1 -> Data Type Conversion/1
  Constant/1 -> Relational Operator/2, Relational Operator1/2, Relational Operator2/2
  S-R Flip-Flop2/1 -> Logical Operator/3
  Relational Operator1/1 -> S-R Flip-Flop1/1
  S-R Flip-Flop/1 -> Logical Operator/1
  S-R Flip-Flop1/1 -> Logical Operator/2
  Relational Operator2/1 -> S-R Flip-Flop2/1
  Demux/1 -> RMS/1
  RMS1/1 -> Relational Operator1/1
  Demux/2 -> RMS1/1
  RMS2/1 -> Relational Operator2/1
  Demux/3 -> RMS2/1

== system 14_bus/Subsystem30/Subsystem1 ==
  Iabc1 : Inport
  Constant : Constant  Value=2  OutDataTypeStr=boolean
  Constant1 : Constant  Value=0  OutDataTypeStr=boolean
  Data Type Conversion : DataTypeConversion  OutDataTypeStr=double  SaturateOnIntegerOverflow=off  RndMeth=Floor
  Demux : Demux  Outputs=3
  Logical Operator : Logic  Inputs=3  AllPortsSameDT=off  OutDataTypeStr=boolean
  RMS : spsRMSLib/RMS  TrueRMS=on  Freq=60  RMSInit=120  Ts=0
  RMS1 : spsRMSLib/RMS  TrueRMS=on  Freq=60  RMSInit=120  Ts=0
  RMS2 : spsRMSLib/RMS  TrueRMS=on  Freq=60  RMSInit=120  Ts=0
  Relational Operator : RelationalOperator  Operator=>  OutDataTypeStr=boolean  RndMeth=Simplest  InputSameDT=off
  Relational Operator1 : RelationalOperator  Operator=>  OutDataTypeStr=boolean  RndMeth=Simplest  InputSameDT=off
  Relational Operator2 : RelationalOperator  Operator=>  OutDataTypeStr=boolean  RndMeth=Simplest  InputSameDT=off
  S-R Flip-Flop : simulink_extras/Flip Flops/S-R Flip-Flop  initial_condition=0
  S-R Flip-Flop1 : simulink_extras/Flip Flops/S-R Flip-Flop  initial_condition=0
  S-R Flip-Flop2 : simulink_extras/Flip Flops/S-R Flip-Flop  initial_condition=0
  Terminator : Terminator
  Terminator1 : Terminator
  Terminator2 : Terminator
  Out1 : Outport
  wires:
  Data Type Conversion/1 -> Out1/1
  Relational Operator/1 -> S-R Flip-Flop/1
  Constant1/1 -> S-R Flip-Flop/2, S-R Flip-Flop1/2, S-R Flip-Flop2/2
  RMS/1 -> Relational Operator/1
  S-R Flip-Flop1/2 -> Terminator1/1
  S-R Flip-Flop/2 -> Terminator/1
  S-R Flip-Flop2/2 -> Terminator2/1
  Iabc1/1 -> Demux/1
  Logical Operator/1 -> Data Type Conversion/1
  Constant/1 -> Relational Operator/2, Relational Operator1/2, Relational Operator2/2
  S-R Flip-Flop2/1 -> Logical Operator/3
  Relational Operator1/1 -> S-R Flip-Flop1/1
  S-R Flip-Flop/1 -> Logical Operator/1
  S-R Flip-Flop1/1 -> Logical Operator/2
  Relational Operator2/1 -> S-R Flip-Flop2/1
  Demux/1 -> RMS/1
  RMS2/1 -> Relational Operator1/1
  Demux/2 -> RMS2/1
  RMS1/1 -> Relational Operator2/1
  Demux/3 -> RMS1/1

== system 14_bus/Subsystem31/Subsystem1 ==
  Iabc1 : Inport
  Constant : Constant  Value=2  OutDataTypeStr=boolean
  Constant1 : Constant  Value=0  OutDataTypeStr=boolean
  Data Type Conversion : DataTypeConversion  OutDataTypeStr=double  SaturateOnIntegerOverflow=off  RndMeth=Floor
  Demux : Demux  Outputs=3
  Logical Operator : Logic  Inputs=3  AllPortsSameDT=off  OutDataTypeStr=boolean
  RMS : spsRMSLib/RMS  TrueRMS=on  Freq=60  RMSInit=120  Ts=0
  RMS1 : spsRMSLib/RMS  TrueRMS=on  Freq=60  RMSInit=120  Ts=0
  RMS2 : spsRMSLib/RMS  TrueRMS=on  Freq=60  RMSInit=120  Ts=0
  Relational Operator : RelationalOperator  Operator=>  OutDataTypeStr=boolean  RndMeth=Simplest  InputSameDT=off
  Relational Operator1 : RelationalOperator  Operator=>  OutDataTypeStr=boolean  RndMeth=Simplest  InputSameDT=off
  Relational Operator2 : RelationalOperator  Operator=>  OutDataTypeStr=boolean  RndMeth=Simplest  InputSameDT=off
  S-R Flip-Flop : simulink_extras/Flip Flops/S-R Flip-Flop  initial_condition=0
  S-R Flip-Flop1 : simulink_extras/Flip Flops/S-R Flip-Flop  initial_condition=0
  S-R Flip-Flop2 : simulink_extras/Flip Flops/S-R Flip-Flop  initial_condition=0
  Terminator : Terminator
  Terminator1 : Terminator
  Terminator2 : Terminator
  Out1 : Outport
  wires:
  Data Type Conversion/1 -> Out1/1
  Relational Operator/1 -> S-R Flip-Flop/1
  Constant1/1 -> S-R Flip-Flop/2, S-R Flip-Flop1/2, S-R Flip-Flop2/2
  RMS1/1 -> Relational Operator/1
  S-R Flip-Flop1/2 -> Terminator1/1
  S-R Flip-Flop/2 -> Terminator/1
  S-R Flip-Flop2/2 -> Terminator2/1
  Iabc1/1 -> Demux/1
  Logical Operator/1 -> Data Type Conversion/1
  Constant/1 -> Relational Operator/2, Relational Operator1/2, Relational Operator2/2
  S-R Flip-Flop2/1 -> Logical Operator/3
  Relational Operator1/1 -> S-R Flip-Flop1/1
  S-R Flip-Flop/1 -> Logical Operator/1
  S-R Flip-Flop1/1 -> Logical Operator/2
  Relational Operator2/1 -> S-R Flip-Flop2/1
  Demux/1 -> RMS1/1
  RMS2/1 -> Relational Operator1/1
  Demux/2 -> RMS2/1
  RMS/1 -> Relational Operator2/1
  Demux/3 -> RMS/1

== system 14_bus/Subsystem32/Subsystem1 ==
  Iabc1 : Inport
  Constant : Constant  Value=2  OutDataTypeStr=boolean
  Constant1 : Constant  Value=0  OutDataTypeStr=boolean
  Data Type Conversion : DataTypeConversion  OutDataTypeStr=double  SaturateOnIntegerOverflow=off  RndMeth=Floor
  Demux : Demux  Outputs=3
  Logical Operator : Logic  Inputs=3  AllPortsSameDT=off  OutDataTypeStr=boolean
  RMS : spsRMSLib/RMS  TrueRMS=on  Freq=60  RMSInit=120  Ts=0
  RMS1 : spsRMSLib/RMS  TrueRMS=on  Freq=60  RMSInit=120  Ts=0
  RMS2 : spsRMSLib/RMS  TrueRMS=on  Freq=60  RMSInit=120  Ts=0
  Relational Operator : RelationalOperator  Operator=>  OutDataTypeStr=boolean  RndMeth=Simplest  InputSameDT=off
  Relational Operator1 : RelationalOperator  Operator=>  OutDataTypeStr=boolean  RndMeth=Simplest  InputSameDT=off
  Relational Operator2 : RelationalOperator  Operator=>  OutDataTypeStr=boolean  RndMeth=Simplest  InputSameDT=off
  S-R Flip-Flop : simulink_extras/Flip Flops/S-R Flip-Flop  initial_condition=0
  S-R Flip-Flop1 : simulink_extras/Flip Flops/S-R Flip-Flop  initial_condition=0
  S-R Flip-Flop2 : simulink_extras/Flip Flops/S-R Flip-Flop  initial_condition=0
  Terminator : Terminator
  Terminator1 : Terminator
  Terminator2 : Terminator
  Out1 : Outport
  wires:
  Data Type Conversion/1 -> Out1/1
  Relational Operator/1 -> S-R Flip-Flop/1
  Constant1/1 -> S-R Flip-Flop/2, S-R Flip-Flop1/2, S-R Flip-Flop2/2
  RMS/1 -> Relational Operator/1
  S-R Flip-Flop1/2 -> Terminator1/1
  S-R Flip-Flop/2 -> Terminator/1
  S-R Flip-Flop2/2 -> Terminator2/1
  Iabc1/1 -> Demux/1
  Logical Operator/1 -> Data Type Conversion/1
  Constant/1 -> Relational Operator/2, Relational Operator1/2, Relational Operator2/2
  S-R Flip-Flop2/1 -> Logical Operator/3
  Relational Operator1/1 -> S-R Flip-Flop1/1
  S-R Flip-Flop/1 -> Logical Operator/1
  S-R Flip-Flop1/1 -> Logical Operator/2
  Relational Operator2/1 -> S-R Flip-Flop2/1
  Demux/1 -> RMS/1
  RMS2/1 -> Relational Operator1/1
  Demux/2 -> RMS2/1
  RMS1/1 -> Relational Operator2/1
  Demux/3 -> RMS1/1

== system 14_bus/Subsystem33/Subsystem1 ==
  Iabc1 : Inport
  Constant : Constant  Value=2  OutDataTypeStr=boolean
  Constant1 : Constant  Value=0  OutDataTypeStr=boolean
  Data Type Conversion : DataTypeConversion  OutDataTypeStr=double  SaturateOnIntegerOverflow=off  RndMeth=Floor
  Demux : Demux  Outputs=3
  Logical Operator : Logic  Inputs=3  AllPortsSameDT=off  OutDataTypeStr=boolean
  RMS : spsRMSLib/RMS  TrueRMS=on  Freq=60  RMSInit=120  Ts=0
  RMS1 : spsRMSLib/RMS  TrueRMS=on  Freq=60  RMSInit=120  Ts=0
  RMS2 : spsRMSLib/RMS  TrueRMS=on  Freq=60  RMSInit=120  Ts=0
  Relational Operator : RelationalOperator  Operator=>  OutDataTypeStr=boolean  RndMeth=Simplest  InputSameDT=off
  Relational Operator1 : RelationalOperator  Operator=>  OutDataTypeStr=boolean  RndMeth=Simplest  InputSameDT=off
  Relational Operator2 : RelationalOperator  Operator=>  OutDataTypeStr=boolean  RndMeth=Simplest  InputSameDT=off
  S-R Flip-Flop : simulink_extras/Flip Flops/S-R Flip-Flop  initial_condition=0
  S-R Flip-Flop1 : simulink_extras/Flip Flops/S-R Flip-Flop  initial_condition=0
  S-R Flip-Flop2 : simulink_extras/Flip Flops/S-R Flip-Flop  initial_condition=0
  Terminator : Terminator
  Terminator1 : Terminator
  Terminator2 : Terminator
  Out1 : Outport
  wires:
  Data Type Conversion/1 -> Out1/1
  Relational Operator/1 -> S-R Flip-Flop/1
  Constant1/1 -> S-R Flip-Flop/2, S-R Flip-Flop1/2, S-R Flip-Flop2/2
  RMS/1 -> Relational Operator/1
  S-R Flip-Flop1/2 -> Terminator1/1
  S-R Flip-Flop/2 -> Terminator/1
  S-R Flip-Flop2/2 -> Terminator2/1
  Iabc1/1 -> Demux/1
  Logical Operator/1 -> Data Type Conversion/1
  Constant/1 -> Relational Operator/2, Relational Operator1/2, Relational Operator2/2
  S-R Flip-Flop2/1 -> Logical Operator/3
  Relational Operator1/1 -> S-R Flip-Flop1/1
  S-R Flip-Flop/1 -> Logical Operator/1
  S-R Flip-Flop1/1 -> Logical Operator/2
  Relational Operator2/1 -> S-R Flip-Flop2/1
  Demux/1 -> RMS/1
  RMS1/1 -> Relational Operator1/1
  Demux/2 -> RMS1/1
  RMS2/1 -> Relational Operator2/1
  Demux/3 -> RMS2/1

== system 14_bus/Subsystem34/Subsystem1 ==
  Iabc1 : Inport
  Constant : Constant  Value=2  OutDataTypeStr=boolean
  Constant1 : Constant  Value=0  OutDataTypeStr=boolean
  Data Type Conversion : DataTypeConversion  OutDataTypeStr=double  SaturateOnIntegerOverflow=off  RndMeth=Floor
  Demux : Demux  Outputs=3
  Logical Operator : Logic  Inputs=3  AllPortsSameDT=off  OutDataTypeStr=boolean
  RMS : spsRMSLib/RMS  TrueRMS=on  Freq=60  RMSInit=120  Ts=0
  RMS1 : spsRMSLib/RMS  TrueRMS=on  Freq=60  RMSInit=120  Ts=0
  RMS2 : spsRMSLib/RMS  TrueRMS=on  Freq=60  RMSInit=120  Ts=0
  Relational Operator : RelationalOperator  Operator=>  OutDataTypeStr=boolean  RndMeth=Simplest  InputSameDT=off
  Relational Operator1 : RelationalOperator  Operator=>  OutDataTypeStr=boolean  RndMeth=Simplest  InputSameDT=off
  Relational Operator2 : RelationalOperator  Operator=>  OutDataTypeStr=boolean  RndMeth=Simplest  InputSameDT=off
  S-R Flip-Flop : simulink_extras/Flip Flops/S-R Flip-Flop  initial_condition=0
  S-R Flip-Flop1 : simulink_extras/Flip Flops/S-R Flip-Flop  initial_condition=0
  S-R Flip-Flop2 : simulink_extras/Flip Flops/S-R Flip-Flop  initial_condition=0
  Terminator : Terminator
  Terminator1 : Terminator
  Terminator2 : Terminator
  Out1 : Outport
  wires:
  Data Type Conversion/1 -> Out1/1
  Relational Operator/1 -> S-R Flip-Flop/1
  Constant1/1 -> S-R Flip-Flop/2, S-R Flip-Flop1/2, S-R Flip-Flop2/2
  RMS/1 -> Relational Operator/1
  S-R Flip-Flop1/2 -> Terminator1/1
  S-R Flip-Flop/2 -> Terminator/1
  S-R Flip-Flop2/2 -> Terminator2/1
  Iabc1/1 -> Demux/1
  Logical Operator/1 -> Data Type Conversion/1
  Constant/1 -> Relational Operator/2, Relational Operator1/2, Relational Operator2/2
  S-R Flip-Flop2/1 -> Logical Operator/3
  Relational Operator1/1 -> S-R Flip-Flop1/1
  S-R Flip-Flop/1 -> Logical Operator/1
  S-R Flip-Flop1/1 -> Logical Operator/2
  Relational Operator2/1 -> S-R Flip-Flop2/1
  Demux/1 -> RMS/1
  RMS1/1 -> Relational Operator1/1
  Demux/2 -> RMS1/1
  RMS2/1 -> Relational Operator2/1
  Demux/3 -> RMS2/1

== system 14_bus/Subsystem35/Subsystem1 ==
  Iabc1 : Inport
  Constant : Constant  Value=2  OutDataTypeStr=boolean
  Constant1 : Constant  Value=0  OutDataTypeStr=boolean
  Data Type Conversion : DataTypeConversion  OutDataTypeStr=double  SaturateOnIntegerOverflow=off  RndMeth=Floor
  Demux : Demux  Outputs=3
  Logical Operator : Logic  Inputs=3  AllPortsSameDT=off  OutDataTypeStr=boolean
  RMS : spsRMSLib/RMS  TrueRMS=on  Freq=60  RMSInit=120  Ts=0
  RMS1 : spsRMSLib/RMS  TrueRMS=on  Freq=60  RMSInit=120  Ts=0
  RMS2 : spsRMSLib/RMS  TrueRMS=on  Freq=60  RMSInit=120  Ts=0
  Relational Operator : RelationalOperator  Operator=>  OutDataTypeStr=boolean  RndMeth=Simplest  InputSameDT=off
  Relational Operator1 : RelationalOperator  Operator=>  OutDataTypeStr=boolean  RndMeth=Simplest  InputSameDT=off
  Relational Operator2 : RelationalOperator  Operator=>  OutDataTypeStr=boolean  RndMeth=Simplest  InputSameDT=off
  S-R Flip-Flop : simulink_extras/Flip Flops/S-R Flip-Flop  initial_condition=0
  S-R Flip-Flop1 : simulink_extras/Flip Flops/S-R Flip-Flop  initial_condition=0
  S-R Flip-Flop2 : simulink_extras/Flip Flops/S-R Flip-Flop  initial_condition=0
  Terminator : Terminator
  Terminator1 : Terminator
  Terminator2 : Terminator
  Out1 : Outport
  wires:
  Data Type Conversion/1 -> Out1/1
  Relational Operator/1 -> S-R Flip-Flop/1
  Constant1/1 -> S-R Flip-Flop/2, S-R Flip-Flop1/2, S-R Flip-Flop2/2
  RMS/1 -> Relational Operator/1
  S-R Flip-Flop1/2 -> Terminator1/1
  S-R Flip-Flop/2 -> Terminator/1
  S-R Flip-Flop2/2 -> Terminator2/1
  Iabc1/1 -> Demux/1
  Logical Operator/1 -> Data Type Conversion/1
  Constant/1 -> Relational Operator/2, Relational Operator1/2, Relational Operator2/2
  S-R Flip-Flop2/1 -> Logical Operator/3
  Relational Operator1/1 -> S-R Flip-Flop1/1
  S-R Flip-Flop/1 -> Logical Operator/1
  S-R Flip-Flop1/1 -> Logical Operator/2
  Relational Operator2/1 -> S-R Flip-Flop2/1
  Demux/1 -> RMS/1
  RMS1/1 -> Relational Operator1/1
  Demux/2 -> RMS1/1
  RMS2/1 -> Relational Operator2/1
  Demux/3 -> RMS2/1
